simulink library "SpeedBoundsAndNoiseSlew"  (R2022b)
settings: Solver=VariableStepAuto  StartTime=0.0  StopTime=10.0  RelTol=1e-3
libraries: TuneVar x8
settings Model: Creator=bt1030690  LastModifiedBy=kl13806
settings SolverCC: AlgebraicLoopSolver=TrustRegion
settings DebuggingCC: UnconnectedInputMsg=warning  UnconnectedOutputMsg=warning  UnconnectedLineMsg=warning  SFMachineParentedDataDiag=warning  ArithmeticOperatorsInVariantConditions=warning
settings ModelReferenceCC: EnableRefExpFcnMdlSchedulingChecks=on
settings SFSimCC: SimUseLocalCustomCode=off  CustomCodeUndefinedFunction=UseInterfaceOnly
settings RTWCC: RTWUseLocalCustomCode=off  DLArmComputeVersion=19.05
settings CodeAppCC: StateflowObjectComments=on

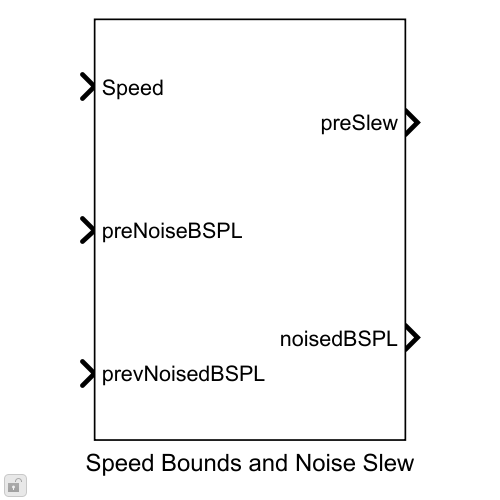
[thumbnail: Simulink's stored preview of the top-level diagram]
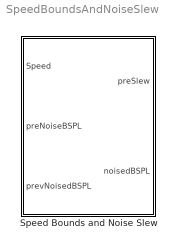
== system SpeedBoundsAndNoiseSlew ==
  Speed Bounds and Noise Slew : Subsystem

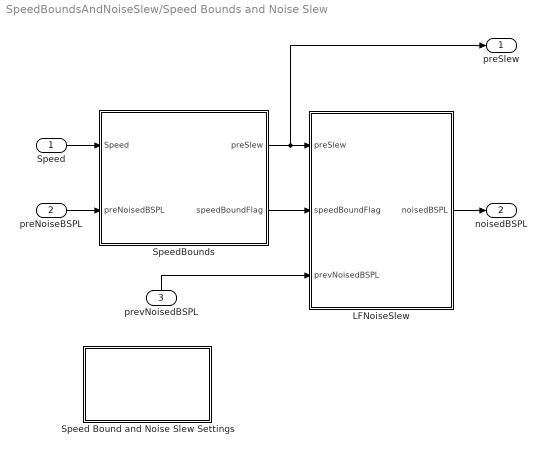
== system SpeedBoundsAndNoiseSlew/Speed Bounds and Noise Slew ==
  Speed : Inport
  preNoiseBSPL : Inport  Port=2
  prevNoisedBSPL : Inport  Port=3
  LFNoiseSlew : Subsystem
  Speed Bound and Noise Slew Settings : Subsystem
  SpeedBounds : Subsystem
  preSlew : Outport  VectorParamsAs1DForOutWhenUnconnected=off
  noisedBSPL : Outport  Port=2  VectorParamsAs1DForOutWhenUnconnected=off
  wires:
  prevNoisedBSPL/1 -> LFNoiseSlew/3(prevNoisedBSPL)
  preNoiseBSPL/1 -> SpeedBounds/2(preNoisedBSPL)
  LFNoiseSlew/1(noisedBSPL) -> noisedBSPL/1
  SpeedBounds/1(preSlew) -> preSlew/1, LFNoiseSlew/1(preSlew)
  SpeedBounds/2(speedBoundFlag) -> LFNoiseSlew/2(speedBoundFlag)
  Speed/1 -> SpeedBounds/1(Speed)

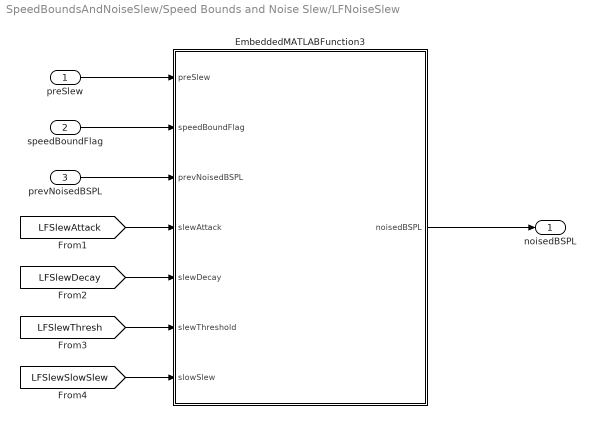
== system SpeedBoundsAndNoiseSlew/Speed Bounds and Noise Slew/LFNoiseSlew ==
  preSlew : Inport
  speedBoundFlag : Inport  Port=2
  prevNoisedBSPL : Inport  Port=3
  EmbeddedMATLABFunction3 : MATLAB Function  TreatAsAtomicUnit=on
  noisedBSPL : Outport  VectorParamsAs1DForOutWhenUnconnected=off
  wires:
  prevNoisedBSPL/1 -> EmbeddedMATLABFunction3/3(prevNoisedBSPL)
  preSlew/1 -> EmbeddedMATLABFunction3/1(preSlew)
  speedBoundFlag/1 -> EmbeddedMATLABFunction3/2(speedBoundFlag)
  EmbeddedMATLABFunction3/1(noisedBSPL) -> noisedBSPL/1
  [LFSlewAttack] -> EmbeddedMATLABFunction3/4(slewAttack)
  [LFSlewDecay] -> EmbeddedMATLABFunction3/5(slewDecay)
  [LFSlewThresh] -> EmbeddedMATLABFunction3/6(slewThreshold)
  [LFSlewSlowSlew] -> EmbeddedMATLABFunction3/7(slowSlew)

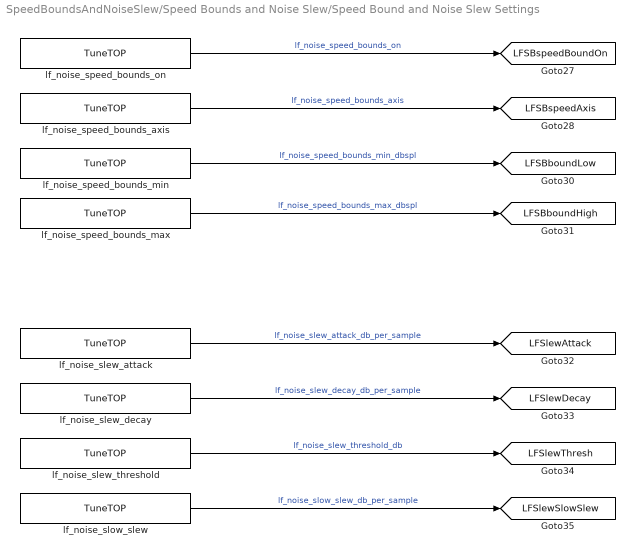
== system SpeedBoundsAndNoiseSlew/Speed Bounds and Noise Slew/Speed Bound and Noise Slew Settings ==
  lf_noise_slew_attack : TuneVar/TuneTOP  TriggerInit=[30 340 200 370]  TopName=lf_noise_slew_attack_db_per_sample  TuneName=lf_noise_slew_attack_db_per_sample  DataType=Inherit: Same as input  PackageName=mode  BankNumber=0  TunabilityNumber=1  MinValue=[]  MaxValue=[]  UseSameName=on  MaskValue=single(LF.Slew.attack)
  lf_noise_slew_decay : TuneVar/TuneTOP  TriggerInit=[30 395 200 425]  TopName=lf_noise_slew_decay_db_per_sample  TuneName=lf_noise_slew_decay_db_per_sample  DataType=Inherit: Same as input  PackageName=mode  BankNumber=0  TunabilityNumber=1  MinValue=[]  MaxValue=[]  UseSameName=on  MaskValue=single(LF.Slew.decay)
  lf_noise_slew_threshold : TuneVar/TuneTOP  TriggerInit=[30 450 200 480]  TopName=lf_noise_slew_threshold_db  TuneName=lf_noise_slew_threshold_db  DataType=Inherit: Same as input  PackageName=mode  BankNumber=0  TunabilityNumber=1  MinValue=[]  MaxValue=[]  UseSameName=on  MaskValue=single([LF.Slew.thresh])
  lf_noise_slow_slew : TuneVar/TuneTOP  TriggerInit=[30 505 200 535]  TopName=lf_noise_slow_slew_db_per_sample  TuneName=lf_noise_slow_slew_db_per_sample  DataType=Inherit: Same as input  PackageName=mode  BankNumber=0  TunabilityNumber=1  MinValue=[]  MaxValue=[]  UseSameName=on  MaskValue=single([LF.Slew.slowSlew])
  lf_noise_speed_bounds_axis : TuneVar/TuneTOP  TriggerInit=[30 105 200 135]  TopName=lf_noise_speed_bounds_axis  TuneName=lf_noise_speed_bounds_axis  DataType=Inherit: Same as input  PackageName=mode  BankNumber=0  TunabilityNumber=1  MinValue=[]  MaxValue=[]  UseSameName=on  MaskValue=single(LF.SB.speedAxis)
  lf_noise_speed_bounds_max : TuneVar/TuneTOP  TriggerInit=[30 210 200 240]  TopName=lf_noise_speed_bounds_max_dbspl  TuneName=lf_noise_speed_bounds_max_dbspl  DataType=Inherit: Same as input  PackageName=mode  BankNumber=0  TunabilityNumber=1  MinValue=[]  MaxValue=[]  UseSameName=on  MaskValue=single(LF.SB.boundHigh)
  lf_noise_speed_bounds_min : TuneVar/TuneTOP  TriggerInit=[30 160 200 190]  TopName=lf_noise_speed_bounds_min_dbspl  TuneName=lf_noise_speed_bounds_min_dbspl  DataType=Inherit: Same as input  PackageName=mode  BankNumber=0  TunabilityNumber=1  MinValue=[]  MaxValue=[]  UseSameName=on  MaskValue=single(LF.SB.boundLow)
  lf_noise_speed_bounds_on : TuneVar/TuneTOP  TriggerInit=[30 50 200 80]  TopName=lf_noise_speed_bounds_on  TuneName=lf_noise_speed_bounds_on  DataType=Inherit: Same as input  PackageName=mode  BankNumber=0  TunabilityNumber=1  MinValue=[]  MaxValue=[]  UseSameName=on  MaskValue=single(1)
  tag scope: LFSBboundHigh=global, LFSBboundLow=global, LFSBspeedAxis=global, LFSBspeedBoundOn=global, LFSlewAttack=global, LFSlewDecay=global, LFSlewSlowSlew=global, LFSlewThresh=global
  wires:
  lf_noise_speed_bounds_max/1 -> [LFSBboundHigh]  "lf_noise_speed_bounds_max_dbspl"
  lf_noise_speed_bounds_min/1 -> [LFSBboundLow]  "lf_noise_speed_bounds_min_dbspl"
  lf_noise_speed_bounds_axis/1 -> [LFSBspeedAxis]  "lf_noise_speed_bounds_axis"
  lf_noise_speed_bounds_on/1 -> [LFSBspeedBoundOn]  "lf_noise_speed_bounds_on"
  lf_noise_slow_slew/1 -> [LFSlewSlowSlew]  "lf_noise_slow_slew_db_per_sample"
  lf_noise_slew_decay/1 -> [LFSlewDecay]  "lf_noise_slew_decay_db_per_sample"
  lf_noise_slew_attack/1 -> [LFSlewAttack]  "lf_noise_slew_attack_db_per_sample"
  lf_noise_slew_threshold/1 -> [LFSlewThresh]  "lf_noise_slew_threshold_db"

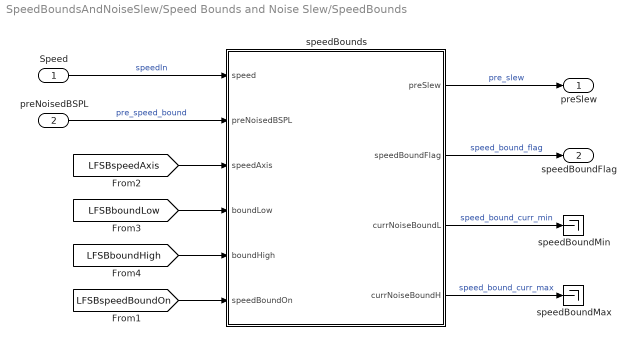
== system SpeedBoundsAndNoiseSlew/Speed Bounds and Noise Slew/SpeedBounds ==
  Speed : Inport
  preNoisedBSPL : Inport  Port=2
  speedBoundMax : Terminator
  speedBoundMin : Terminator
  speedBounds : MATLAB Function  TreatAsAtomicUnit=on
  preSlew : Outport  VectorParamsAs1DForOutWhenUnconnected=off
  speedBoundFlag : Outport  Port=2  VectorParamsAs1DForOutWhenUnconnected=off
  wires:
  speedBounds/2(speedBoundFlag) -> speedBoundFlag/1  "speed_bound_flag"
  speedBounds/1(preSlew) -> preSlew/1  "pre_slew"
  preNoisedBSPL/1 -> speedBounds/2(preNoisedBSPL)  "pre_speed_bound"
  Speed/1 -> speedBounds/1(speed)  "speedIn"
  [LFSBspeedAxis] -> speedBounds/3(speedAxis)
  [LFSBspeedBoundOn] -> speedBounds/6(speedBoundOn)
  [LFSBboundLow] -> speedBounds/4(boundLow)
  [LFSBboundHigh] -> speedBounds/5(boundHigh)
  speedBounds/3(currNoiseBoundL) -> speedBoundMin/1  "speed_bound_curr_min"
  speedBounds/4(currNoiseBoundH) -> speedBoundMax/1  "speed_bound_curr_max"

== matlab function SpeedBoundsAndNoiseSlew/Speed Bounds and Noise Slew/SpeedBounds/speedBounds ==
  data: speed input; preNoisedBSPL input size=1; speedAxis input; boundLow input; boundHigh input; speedBoundOn input; preSlew output; speedBoundFlag output; currNoiseBoundL output; currNoiseBoundH output
function [preSlew, speedBoundFlag, currNoiseBoundL, currNoiseBoundH] ...
    = speedBounds(speed, preNoisedBSPL, ...
        speedAxis, boundLow, boundHigh, speedBoundOn)
% Initialize the varibales based on the speedBoundOn value
if speedBoundOn > 0
	currNoiseBoundL = interp1(speedAxis, boundLow, speed, 'linear');
	currNoiseBoundH = interp1(speedAxis, boundHigh, speed, 'linear');
	preSlew = single(max(preNoisedBSPL, currNoiseBoundL));
	preSlew = single(min(preSlew, currNoiseBoundH));
	% Check whether preSlew not equal preNoisedBSPL
	if (preSlew ~= preNoisedBSPL)
		speedBoundFlag = 1;% If not Equal then Enable the flag
	else
		speedBoundFlag = 0;% If Equal Disable the flag
	end
else
	preSlew = single(preNoisedBSPL);
	speedBoundFlag = 0; % Assign Zero
    currNoiseBoundL = single(0); % Assign Zero
    currNoiseBoundH = single(0); % Assign Zero
end
end

== matlab function SpeedBoundsAndNoiseSlew/Speed Bounds and Noise Slew/LFNoiseSlew/EmbeddedMATLABFunction3 ==
  data: preSlew input size=1; speedBoundFlag input; prevNoisedBSPL input; slewAttack input =slewAttack; slewDecay input =slewDecay; slewThreshold input =slewThreshold; slowSlew input size=1 =slowSlew; noisedBSPL output
function noisedBSPL = noiseSlew(preSlew, speedBoundFlag, prevNoisedBSPL, ...
	slewAttack, slewDecay, slewThreshold, slowSlew)
	
persistent prevChange prevDelta;
if isempty(prevChange); prevChange = single(0);  end
if isempty(prevDelta); prevDelta = single(0);  end

delta = preSlew - prevNoisedBSPL;

if delta > 0                              % setup for positive delta
	change = min(slewAttack, delta);
	slowSlew = min(slowSlew, delta);
else                                      % setup for negative delta
	change = max(slewDecay, delta);
	slowSlew = max(-slowSlew, delta);
end

if prevDelta*delta > 0					  % did we reach our target?
	slew = single(prevChange);                    % no, continue the current path
else                                      % otherwise, we have reached our target
	slew = single(0);                             % no slew in the dead zone
end

if speedBoundFlag && slew == 0            % are we speed-bounded?
	slew = slowSlew;                      % yes, change to a slow slew
end

if (abs(delta) <= slewThreshold) ...		% are we within the zone?
		&& (abs(slew) < abs(change))          % is change still bigger than slew?
	% (offshoot protection)x
	change = slew;                        % freeze or continue the current
end

prevDelta = delta;
prevChange = change;

prevNoisedBSPL = prevNoisedBSPL + change;
noisedBSPL = prevNoisedBSPL;
end
